simulink model "turbo_code_punc"  (Simulink 7.7)
settings: Solver=VariableStepDiscrete  StartTime=0.0  StopTime=8  FixedStep=Auto  RelTol=1e-3
PostLoadFcn:
  | turbo_code_punc_setup;
values from neighbouring files (symbols this model uses):
  Iter = 6    [turbo_code_no_punc_multiple_run_driver.m]    (also in turbo_code_punc_multiple_run_driver.m)
  Len = 512*512    (= 262144)    [turbo_code_no_punc_multiple_run_driver.m]    (also in turbo_code_punc_multiple_run_driver.m)
  Variance = Ps*multiplier/EsNo    [turbo_code_no_punc_multiple_run_driver.m]    (also in turbo_code_punc_multiple_run_driver.m)
undefined symbols (not defined in the file or in its folder): Max
libraries: commsequence2 x6, commblkintrlv2 x6, commcnvcod2 x4, commchan3 x1, commrandsrc2 x1, commsink2 x1, dspstat3 x1, dspsrcs4 x1, dspindex x1, dspsigops x1, commutil2 x1
Description:
  | a turbo code
  | 1/2 code rate, with puncturing
  | 
  | generator polynomials
  | G =[1 1 1 1 1
  |         1 0 0 0 1]
  | 
  | Reference:  Digital Communications, 2nd edition, B. Sklar,
  |                         2001, Prentice Hall
  |                         pp. 496-497.
settings Model: Creator=In Soo Ahn  LastModifiedBy=isa
settings Model: ModifiedHistory=|
  | Your comments and suggestions are welcome.
  | isa@bradley.edu
settings SolverCC: ConsecutiveZCsStepRelTol=1*128*eps
settings OptimizationCC: InitFltsAndDblsToZero=on
settings DebuggingCC: SaveWithParameterizedLinksMsg=none  SignalResolutionControl=TryResolveAllWithWarning  DiscreteInheritContinuousMsg=error  MultiTaskDSMMsg=warning  MultiTaskCondExecSysMsg=none  StrictBusMsg=Warning
settings RTWCC: IncludeERTFirstTime=on
settings GRTTargetCC: TargetFcnLib=ansi_tfl_tmw.mat

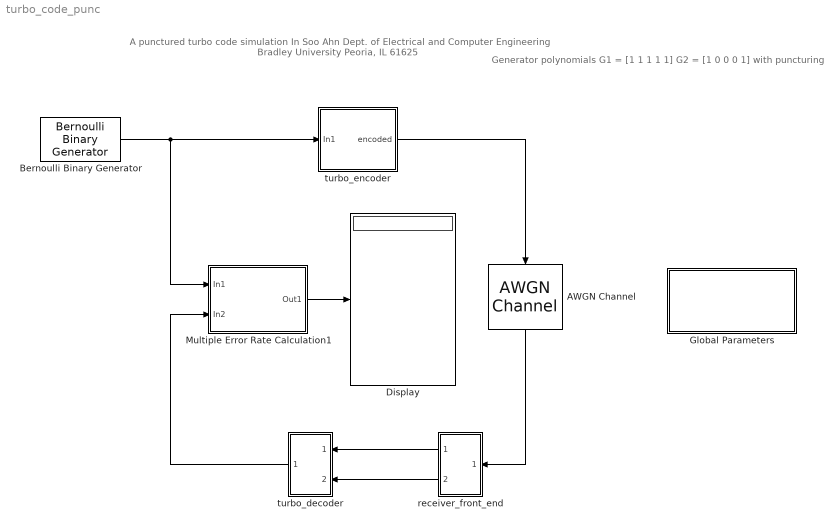
== system turbo_code_punc ==
  note: A punctured turbo code simulation
      | In Soo Ahn
      | Dept. of Electrical and Computer Engineering
      | Bradley University
      | Peoria, IL 61625
  note: Generator polynomials
      | G1 = [1 1 1 1 1]
      | G2 = [1 0 0 0 1]
      | with puncturing
  AWGN Channel : commchan3/AWGN Channel  SystemSampleTime=-1  InputProcessing=Inherited (this choice will be removed - see release notes)  seed=1  noiseMode=Variance from mask  EbNodB=2  EsNodB=10  SNRdB=10  bitsPerSym=2  Ps=1  Tsym=Iter/Len  variance=Variance
  Bernoulli Binary Generator : commrandsrc2/Bernoulli Binary Generator  SystemSampleTime=-1  P=0.5  seed=61  Ts=1  frameBased=on  sampPerFrame=Len  orient=off  outDataType=boolean
  Display : Display
  Global Parameters : Subsystem  mask(Global Parameters){EbNodB=1.6, Len=256*256*32, Iter=8, Seed=54123}
      mask prompts: EbNodB "Eb/No in dB:"; Len "Block size:"; Iter "Number of iterations:"
      mask help: Load global parameters in MATLAB workspace.
      mask init:
      | turbo_code_punc_setup;
      mask CallbackString: turbo_code_setup;|turbo_code_setup|turbo_code_setup;|turbo_code_setup;
      mask Display: disp(['Eb/No ' num2str(EbNodB,'%3.1f') 'dB'  sprintf('\n') 'Block size   ' num2str(Len,'%7.0f')  sprintf('\n') 'Iterations   ' num2str(Iter,'%3.0f')   sprintf('\n') 'Seed   ' num2str(Seed,'%7.0f')])
  Multiple Error Rate Calculation1 : Subsystem
      mask Display: disp('Multiple\nIteration\nError Rate\nCalculation')
  receiver_front_end : Subsystem
  turbo_decoder : Subsystem
  turbo_encoder : Subsystem
  wires:
  Multiple Error Rate Calculation1/1(Out1) -> Display/1
  turbo_decoder/1(Out1) -> Multiple Error Rate Calculation1/2(In2)
  Bernoulli Binary Generator/1 -> turbo_encoder/1(In1), Multiple Error Rate Calculation1/1(In1)
  receiver_front_end/1(Out1) -> turbo_decoder/1(In1)
  receiver_front_end/2(Out2) -> turbo_decoder/2(In2)
  turbo_encoder/1(encoded) -> AWGN Channel/1
  AWGN Channel/1 -> receiver_front_end/1(In1)

== system turbo_code_punc/Global Parameters ==

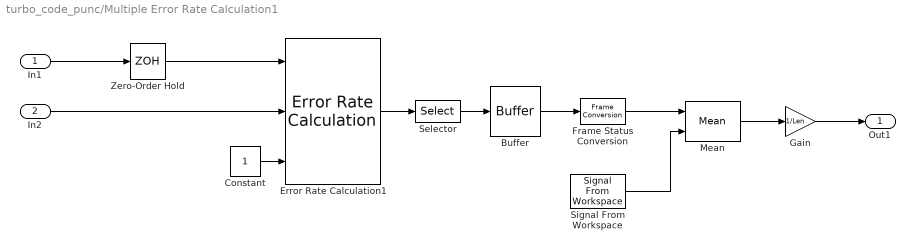
== system turbo_code_punc/Multiple Error Rate Calculation1 ==
  In1 : Inport
  In2 : Inport  Port=2
  Buffer : Buffer  N=Iter
  Constant : Constant
  Error Rate Calculation1 : commsink2/Error Rate Calculation  N=0  st_delay=0  cp_mode=Entire frame  subframe=[]  PMode=Port  WsName=ErrorVec1  RsMode2=on  stop=off  numErr=100  maxBits=1e6
  Frame Status Conversion : FrameConversion  OutFrame=Sample-based
  Gain : Gain  Gain=1/Len  SaturateOnIntegerOverflow=on  OutDataTypeStr=Inherit: Same as input  ParamDataTypeStr=Inherit: Same as input
  Mean : dspstat3/Mean  run=on  reset_popup=Non-zero sample  InputProcessing=Inherited (this choice will be removed - see release notes)  directionMode=Each column  dimension=1  treatSBRowAsCol=on  roiEnable=off  roiType=Rectangles  roiPortion=Entire ROI  roiOutput=Individual statistics for each ROI  roiFlag=off  outputDataTypeStr=Inherit: Same as accumulator  outputLastDataTypeStr=Inherit: Same as accumulator  outputMin=[]  outputMax=[]  roundingMode=Floor  overflowMode=off
  Selector : Selector  InputPortWidth=3  IndexOptions=Index vector (dialog)  Indices=2  OutputSizes=1
  Signal From Workspace : dspsrcs4/Signal From Workspace  SystemSampleTime=-1  X=[1 1]  Ts=Iter  nsamps=1  OutputAfterFinalValue=Setting to zero  ignoreOrWarnInputAndFrameLengths=off
  Zero-Order Hold : ZeroOrderHold
  Out1 : Outport
  wires:
  In1/1 -> Zero-Order Hold/1
  Error Rate Calculation1/1 -> Selector/1
  Selector/1 -> Buffer/1
  In2/1 -> Error Rate Calculation1/2
  Buffer/1 -> Frame Status Conversion/1
  Frame Status Conversion/1 -> Mean/1
  Zero-Order Hold/1 -> Error Rate Calculation1/1
  Constant/1 -> Error Rate Calculation1/3
  Mean/1 -> Gain/1
  Gain/1 -> Out1/1
  Signal From Workspace/1 -> Mean/2

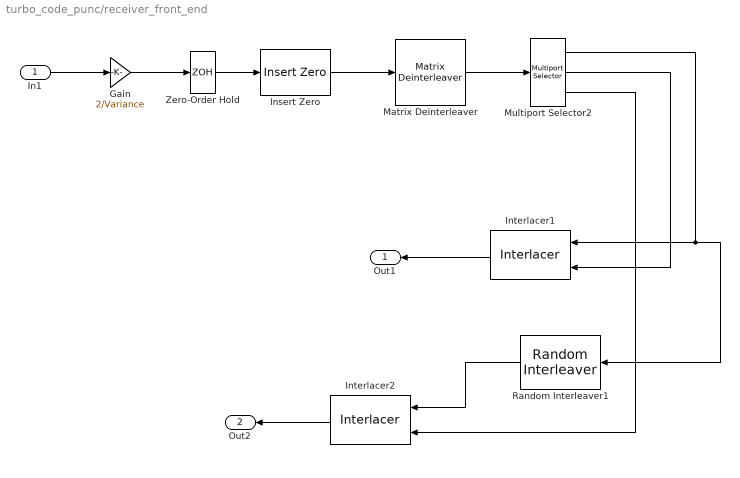
== system turbo_code_punc/receiver_front_end ==
  In1 : Inport
  Gain : Gain  Gain=2/Variance  SampleTime=1
  Insert Zero : commsequence2/Insert Zero  insertZeroVector=[1 1 0 1 0 1].'
  Interlacer1 : commsequence2/Interlacer
  Interlacer2 : commsequence2/Interlacer
  Matrix Deinterleaver : commblkintrlv2/Matrix Deinterleaver  SystemSampleTime=-1  Nrows=3  Ncols=Len
  Multiport Selector2 : dspindex/Multiport Selector  rowsOrCols=Rows  idxCellArray={1:Len, Len+1:2*Len, 2*Len+1:3*Len}  idxErrMode=Clip Index
  Random Interleaver1 : commblkintrlv2/Random Interleaver  SystemSampleTime=-1  N=Len  seed=Seed
  Zero-Order Hold : ZeroOrderHold  SampleTime=Iter
  Out1 : Outport
  Out2 : Outport  Port=2
  wires:
  Multiport Selector2/1 -> Interlacer1/1, Random Interleaver1/1
  Multiport Selector2/2 -> Interlacer1/2
  Random Interleaver1/1 -> Interlacer2/1
  Multiport Selector2/3 -> Interlacer2/2
  Zero-Order Hold/1 -> Insert Zero/1
  In1/1 -> Gain/1
  Interlacer1/1 -> Out1/1
  Interlacer2/1 -> Out2/1
  Matrix Deinterleaver/1 -> Multiport Selector2/1
  Insert Zero/1 -> Matrix Deinterleaver/1
  Gain/1 -> Zero-Order Hold/1

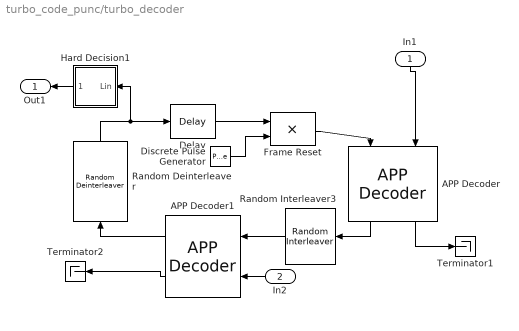
== system turbo_code_punc/turbo_decoder ==
  In1 : Inport
  In2 : Inport  Port=2
  APP Decoder : commcnvcod2/APP Decoder  trellis=trellis  termMethod=Truncated  algorithm=Max*  maxStarNumScaleBits=3
  APP Decoder1 : commcnvcod2/APP Decoder  trellis=trellis  termMethod=Truncated  algorithm=Max*  maxStarNumScaleBits=3
  Delay : dspsigops/Delay  InputProcessing=Inherited (this choice will be removed - see release notes)  dly_unit=Samples  delay=Len  ic_detail=off  dif_ic_for_ch=off  dif_ic_for_dly=off  ic=0  reset_popup=None
  Discrete Pulse Generator : DiscretePulseGenerator  Period=Iter  PulseWidth=Iter-1  PhaseDelay=1
  Frame Reset : Product  SaturateOnIntegerOverflow=on  InputSameDT=on  OutDataTypeStr=Inherit: Same as first input
  Hard Decision1 : Subsystem
      mask Type: Hard Decision
      mask Description: Likelihood to binary transformation.
  Random Deinterleaver : commblkintrlv2/Random Deinterleaver  SystemSampleTime=-1  N=Len  seed=Seed
  Random Interleaver3 : commblkintrlv2/Random Interleaver  SystemSampleTime=-1  N=Len  seed=Seed
  Terminator1 : Terminator
  Terminator2 : Terminator
  Out1 : Outport
  wires:
  APP Decoder1/1 -> Random Deinterleaver/1
  APP Decoder/2 -> Terminator1/1
  APP Decoder1/2 -> Terminator2/1
  Random Deinterleaver/1 -> Delay/1, Hard Decision1/1(Lin)
  Random Interleaver3/1 -> APP Decoder1/1
  APP Decoder/1 -> Random Interleaver3/1
  Frame Reset/1 -> APP Decoder/1
  Delay/1 -> Frame Reset/1
  Discrete Pulse Generator/1 -> Frame Reset/2
  Hard Decision1/1(0/1) -> Out1/1
  In1/1 -> APP Decoder/2
  In2/1 -> APP Decoder1/2

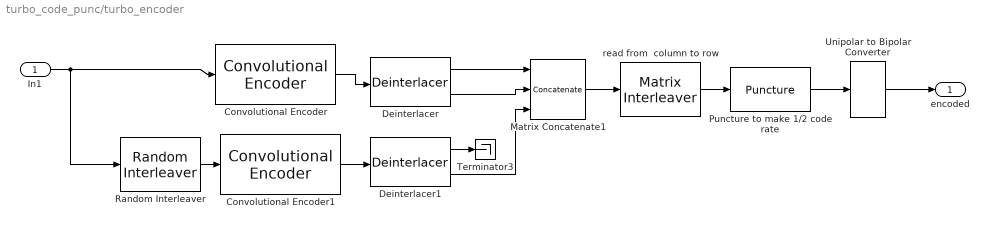
== system turbo_code_punc/turbo_encoder ==
  In1 : Inport
  Convolutional Encoder : commcnvcod2/Convolutional Encoder  trellis=trellis  opMode=Continuous  DelayedResetAction=off  hasIniStPort=off  hasFinStPort=off  usePuncVector=off  punctureVector=[ 1 1 0 1 0 1]'  reset=Unused parameter value
  Convolutional Encoder1 : commcnvcod2/Convolutional Encoder  trellis=trellis  opMode=Truncated (reset every frame)  DelayedResetAction=off  hasIniStPort=off  hasFinStPort=off  usePuncVector=off  punctureVector=[ 1 1 0 1 0 1]'  reset=Unused parameter value
  Deinterlacer : commsequence2/Deinterlacer
  Deinterlacer1 : commsequence2/Deinterlacer
  Matrix Concatenate1 : Concatenate  NumInputs=3  Mode=Multidimensional array
  Puncture to make 1/2 code rate : commsequence2/Puncture  punctureVector=[1 1 0 1 0 1].'
  Random Interleaver : commblkintrlv2/Random Interleaver  SystemSampleTime=-1  N=Len  seed=Seed
  Terminator3 : Terminator
  Unipolar to Bipolar Converter : commutil2/Unipolar to Bipolar Converter  SystemSampleTime=-1  M=2  polarity=Positive  dataType=double
  read from  column to row : commblkintrlv2/Matrix Interleaver  SystemSampleTime=-1  Nrows=3  Ncols=Len
  encoded : Outport
  wires:
  In1/1 -> Convolutional Encoder/1, Random Interleaver/1
  Unipolar to Bipolar Converter/1 -> encoded/1
  Random Interleaver/1 -> Convolutional Encoder1/1
  Convolutional Encoder/1 -> Deinterlacer/1
  Convolutional Encoder1/1 -> Deinterlacer1/1
  Deinterlacer1/1 -> Terminator3/1
  Deinterlacer/1 -> Matrix Concatenate1/1
  Deinterlacer1/2 -> Matrix Concatenate1/3
  read from  column to row/1 -> Puncture to make 1/2 code rate/1
  Matrix Concatenate1/1 -> read from  column to row/1
  Puncture to make 1/2 code rate/1 -> Unipolar to Bipolar Converter/1
  Deinterlacer/2 -> Matrix Concatenate1/2

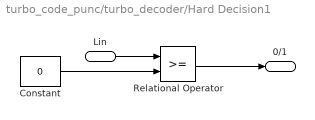
== system turbo_code_punc/turbo_decoder/Hard Decision1 ==
  Lin : Inport
  Constant : Constant  Value=0
  Relational Operator : RelationalOperator  InputSameDT=on
  0/1 : Outport
  wires:
  Constant/1 -> Relational Operator/2
  Lin/1 -> Relational Operator/1
  Relational Operator/1 -> 0/1/1
